simulink model "Dynamics_test"  (R2023b)
settings: Solver=FixedStepAuto  StartTime=0.0  StopTime=30  FixedStep=1e-4  RelTol=1e-3
values from neighbouring files (symbols this model uses):
  aircraft_b = 2    [initial.m]
  aircraft_c = 0.275    [initial.m]
  aircraft_mass = 6.031    [initial.m]
  c1 = ((Iyy - Izz)*Izz - Ixz*Ixz)/sigma    (= -0.404494382022)    [initial.m]
  c2 = ((Ixx - Iyy + Izz)*Ixz)/sigma    (= 0)    [initial.m]
  c3 = Izz/sigma    (= 3.74531835206)    [initial.m]
  c4 = Ixz/sigma    (= 0)    [initial.m]
  c5 = (Izz - Ixx)/Iyy    (= 0.404494382022)    [initial.m]
  c6 = Ixz/Iyy    (= 0)    [initial.m]
  c7 = 1/Iyy    (= 3.74531835206)    [initial.m]
  c8 = (Ixx*(Ixx - Iyy) + Ixz*Ixz)/sigma    (= 0)    [initial.m]
  c9 = Ixx/sigma    (= 2.66666666667)    [initial.m]
  CD_fuselage = 0.027    [initial.m]
  CdDa = 0.092132    [initial.m]
  CdDe = 0.016043    [initial.m]
  CdDr = 0.0097403    [initial.m]
  CDmin = 0.06047    [initial.m]
  CL0 = 0.81857    [initial.m]
  CL_CDmin = 0.4806    [initial.m]
  CLa = 4.09127    [initial.m]
  CLa_dot = 0    [initial.m]
  Clb = -0.00161    [initial.m]
  ClDa = 0.286593    [initial.m]
  CLDa = -0.85291    [initial.m]
  CLDe = 0.50787    [initial.m]
  ClDr = 0.013407    [initial.m]
  Clp = -0.47584    [initial.m]
  CLq = 7.31097    [initial.m]
  Clr = 0.27153    [initial.m]
  Cm0 = 0.00763    [initial.m]
  Cma = -1.76966    [initial.m]
  CmDe = -1.83747    [initial.m]
  Cmq = -19.22663    [initial.m]
  Cnb = 0.0918    [initial.m]
  CnDa = 0.0049274    [initial.m]
  CnDr = -0.067036    [initial.m]
  Cnp = -0.13267    [initial.m]
  Cnr = -0.08829    [initial.m]
  CYb = -0.00157    [initial.m]
  CYDr = 0.128915    [initial.m]
  CYp = -0.00157    [initial.m]
  CYr = 0.18368    [initial.m]
  F_T = C_T*rho*n_trim^2*PropDiameter^4    [initial.m]
  g = 9.8060    (= 9.806)    [initial.m]
  init_aileron = 0    [initial.m]
  init_alpha = alpha_trim    (= 0)    [initial.m]
  init_beta = atan(init_v/init_V)    [initial.m]
  init_elevator = elevator_trim    (= 0)    [initial.m]
  init_h = 10    [initial.m]
  init_p = 0    [initial.m]
  init_phi = 0    [initial.m]
  init_psi = 0    [initial.m]
  init_q = 0    [initial.m]
  init_r = 0    [initial.m]
  init_rudder = 0    [initial.m]
  init_theta = init_alpha    (= 0)    [initial.m]
  init_u = Vb(1)    [initial.m]
  init_v = Vb(2)    [initial.m]
  init_w = Vb(3)    [initial.m]
  init_x = 0    [initial.m]
  init_y = 0    [initial.m]
  K = 0.1328    [initial.m]
  Max_RPM = 10000    [initial.m]
  PropDiameter = 0.3052    [initial.m]
  rho = 1.2250    (= 1.225)    [initial.m]
  rotor1_direction = 1    [initial.m]
  rotor2_direction = -1    [initial.m]
  rotor3_direction = -1    [initial.m]
  rotor4_direction = 1    [initial.m]
  rotor_arm1 = [0.375,0.375,0]    [initial.m]
  rotor_arm2 = [0.375,-0.375,0]    [initial.m]
  rotor_arm3 = [-0.375,-0.375,0]    [initial.m]
  rotor_arm4 = [-0.375,0.375,0]    [initial.m]
  RPM_init = 0    [initial.m]
  tilt1_init = lambda    [initial.m]
  tilt2_init = lambda    [initial.m]
  tilt3_init = 0    [initial.m]
  tilt4_init = 0    [initial.m]
undefined symbols (not defined in the file or in its folder): linmodel, linmodel2
libraries: simulink_extras x14, aerolibasang x5, matrix_library x4
settings Model: Creator=admin  LastModifiedBy=admin

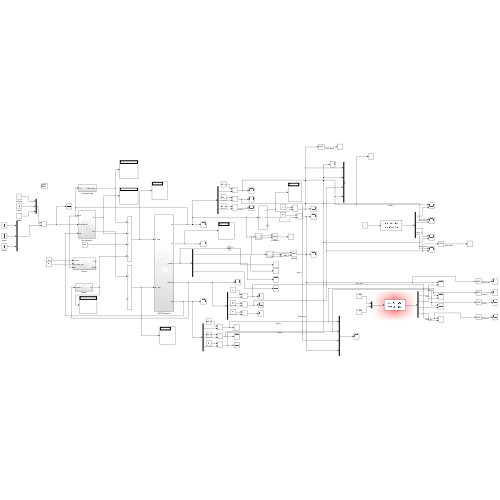
[thumbnail: Simulink's stored preview of the top-level diagram]
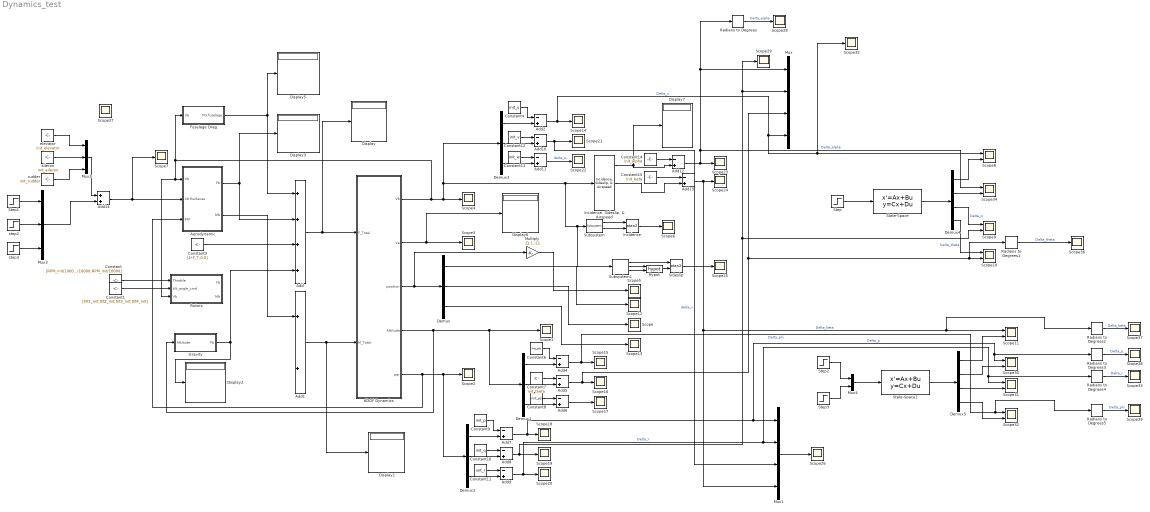
== system Dynamics_test ==
  6DOF Dynamics : Subsystem
  Add : Sum  Inputs=++++
  Add1 : Sum
  Add{2,4..13} (11 alike) : Sum  Inputs=-+
  Add14 : Sum
  Aerodynamic : Subsystem
  Constant : Constant  Value=[RPM_init/10000;RPM_init/10000;RPM_init/10000;RPM_init/10000]
  Constant1 : Constant  Value=[tilt1_init;tilt2_init;tilt3_init;tilt4_init]
  Constant10 : Constant  Value=init_q
  Constant11 : Constant  Value=init_r
  Constant12 : Constant  Value=init_v
  Constant13 : Constant  Value=init_w
  Constant14 : Constant  Value=init_alpha
  Constant15 : Constant  Value=init_beta
  Constant3 : Constant  Value=[4*F_T;0;0]
  Constant4 : Constant  Value=init_u
  Constant6 : Constant  Value=init_phi
  Constant7 : Constant  Value=init_theta
  Constant8 : Constant  Value=init_psi
  Constant9 : Constant  Value=init_p
  Demux{,1..3} (4 alike) : Demux  Outputs=3
  Demux4 : Demux
  Demux5 : Demux
  Display{,1..3,5..7} (7 alike) : Display
  Fuselage Drag : Subsystem
  Gravity : Subsystem
  Hypot : Math  Operator=hypot
  Incidence : Trigonometry  Operator=atan2
  "Incidence, Sideslip, & Airspeed" : aerolibasang/Incidence, Sideslip, & Airspeed
  Multiply : Gain  Gain=[1;1;-1]
  Mux : Mux
  Mux1 : Mux
  Mux2 : Mux  Inputs=3
  Mux3 : Mux  Inputs=3
  Mux4 : Mux  Inputs=2
  Radians to Degrees{,1..5} (6 alike) : simulink_extras/Transformations/Radians to Degrees
  Rotors : Subsystem
  Scope{,1..7,12..29,33,35..39} (32 alike) : Scope
  Scope{8..11,30..32,34} (8 alike) : Scope  NumInputPorts=2
  Sideslip : Trigonometry  Operator=atan2
  State-Space : StateSpace  A=linmodel.A  B=linmodel.B  C=linmodel.C  D=linmodel.D  InitialCondition=[0;0;0;0]
  State-Space1 : StateSpace  A=linmodel2.A  B=linmodel2.B  C=linmodel2.C  D=linmodel2.D  InitialCondition=[0;0;0;0]
  Step{,1..3} (4 alike) : Step  After=0  SampleTime=0
  Subsystem : aerolibasang/Incidence, Sideslip, & Airspeed/Subsystem  SystemSampleTime=-1  VariantActivationTime=update diagram  AllowFlexibleInterface=on  Latency=0  AutoFrameSizeCalculation=off
  Subsystem1 : aerolibasang/Incidence, Sideslip, & Airspeed/Subsystem1  SystemSampleTime=-1  VariantActivationTime=update diagram  AllowFlexibleInterface=on  Latency=0  AutoFrameSizeCalculation=off
  aileron : Constant  Value=init_aileron
  elevator : Constant  Value=init_elevator
  rudder : Constant  Value=init_rudder
  step2 : Step  After=0  SampleTime=0
  step3 : Step  After=deg2rad(1)  SampleTime=0
  wires:
  Add/1 -> 6DOF Dynamics/1(F_Total), Display/1
  Add1/1 -> 6DOF Dynamics/2(M_Total), Display1/1
  6DOF Dynamics/4(Attitude) -> Gravity/1(Attitude), Demux1/1, Scope1/1
  6DOF Dynamics/2(Ve) -> Display6/1, Scope3/1
  Demux/2 -> Scope/1
  Demux/1 -> Scope12/1
  Constant/1 -> Rotors/1(Throttle)
  Aerodynamic/2(Mb) -> Add1/1
  Constant1/1 -> Rotors/2(tilt_angle_cmd)
  Demux/3 -> Scope13/1
  Gravity/1(Fb) -> Add/4, Display2/1
  Aerodynamic/1(Fb) -> Display3/1, Add/2
  Fuselage Drag/1(FD,fuselage) -> Display5/1, Add/1
  6DOF Dynamics/3(position) -> Multiply/1, Demux/1
  Multiply/1 -> Scope5/1
  Constant3/1 -> Add/3
  Demux1/1 -> Add4/2
  Constant6/1 -> Add4/1
  Demux1/2 -> Add5/2
  Constant7/1 -> Add5/1
  Demux1/3 -> Add6/2
  Constant8/1 -> Add6/1
  Add4/1 -> Radians to Degrees5/1, Scope32/1, Scope15/1  "Delta_phi"
  Add5/1 -> Radians to Degrees1/1, Scope10/2, Mux/3, Scope16/1
  Add6/1 -> Scope17/1
  Add9/1 -> Radians to Degrees4/1, Scope31/1, Mux1/2, Scope20/1  "Delta_r"
  Constant11/1 -> Add9/1
  Constant9/1 -> Add7/1
  Add7/1 -> Radians to Degrees3/1, Scope30/1, Mux1/1, Scope18/1  "Delta_p"
  6DOF Dynamics/5(pqr) -> Aerodynamic/3(pqr), Demux2/1, Scope2/1
  Constant10/1 -> Add8/1
  Demux2/2 -> Add8/2
  Demux2/1 -> Add7/2
  Demux2/3 -> Add9/2
  Add11/1 -> Scope22/1  "delta_w"
  Constant13/1 -> Add11/1
  Constant4/1 -> Add2/1
  Add2/1 -> Scope35/1, Scope8/1, Mux/4, Scope14/1  "Delta_u"
  Constant12/1 -> Add10/1
  Demux3/2 -> Add10/2
  Demux3/1 -> Add2/2
  Demux3/3 -> Add11/2
  Constant14/1 -> Add12/1
  Add12/1 -> Scope34/1, Mux/1, Radians to Degrees/1, Scope23/1  "Delta_alpha"
  "Incidence, Sideslip, & Airspeed"/1 -> Display7/1, Add12/2
  Constant15/1 -> Add13/1
  "Incidence, Sideslip, & Airspeed"/2 -> Add13/2
  Add8/1 -> Scope9/2, Mux/2, Scope29/1, Scope19/1
  Add10/1 -> Mux1/3, Scope21/1  "delta_v"
  Add13/1 -> Radians to Degrees2/1, Scope11/1, Mux1/4, Scope24/1  "Delta_beta"
  Mux1/1 -> Scope26/1
  Add14/1 -> Scope7/1, Aerodynamic/2(CtrlSurfaces)
  Mux2/1 -> Add14/1
  rudder/1 -> Mux2/3
  aileron/1 -> Mux2/2
  elevator/1 -> Mux2/1
  Subsystem/2 -> Incidence/2
  Subsystem/1 -> Incidence/1
  Incidence/1 -> Scope6/1
  State-Space/1 -> Demux4/1
  Demux4/1 -> Scope8/2
  Step/1 -> State-Space/1
  step3/1 -> Mux3/3
  step2/1 -> Mux3/2
  Step1/1 -> Mux3/1
  Mux3/1 -> Add14/2
  Demux4/2 -> Scope34/2
  Demux4/3 -> Scope9/1  "Delta_q"
  Demux4/4 -> Scope10/1  "Delta_theta"
  Subsystem1/3 -> Hypot/2
  6DOF Dynamics/1(Vb) -> Fuselage Drag/1(Vb), Rotors/3(Vb), Aerodynamic/1(Vb), Demux3/1, Subsystem1/1, Subsystem/1, "Incidence, Sideslip, & Airspeed"/1, Scope4/1
  Hypot/1 -> Sideslip/2
  Subsystem1/2 -> Hypot/1
  Sideslip/1 -> Scope25/1
  Subsystem1/1 -> Sideslip/1
  State-Space1/1 -> Demux5/1
  Demux5/2 -> Scope30/2
  Demux5/3 -> Scope31/2
  Demux5/4 -> Scope32/2
  Step2/1 -> Mux4/1
  Step3/1 -> Mux4/2
  Mux4/1 -> State-Space1/1
  Demux5/1 -> Scope11/2
  Radians to Degrees/1 -> Scope28/1  "Delta_alpha"
  Radians to Degrees1/1 -> Scope36/1  "Delta_theta"
  Radians to Degrees2/1 -> Scope37/1  "Delta_beta"
  Radians to Degrees3/1 -> Scope38/1  "Delta_p"
  Radians to Degrees4/1 -> Scope33/1  "Delta_r"
  Radians to Degrees5/1 -> Scope39/1  "Delta_phi"

== system Dynamics_test/6DOF Dynamics ==
  F_Total : Inport
  M_Total : Inport  Port=2
  Attitude_Function : Subsystem
  Display : Display
  Force_Function : Subsystem
  Integrator : Integrator  InitialCondition=[init_u;init_v;init_w]
  Integrator1 : Integrator  InitialCondition=[init_phi;init_theta;init_psi]  WrapState=on
  Integrator2 : Integrator  InitialCondition=[init_x;init_y;-init_h]
  Integrator3 : Integrator  InitialCondition=[init_p;init_q;init_r]
  MatrixMultiply : Product  Multiplication=Matrix(*)
  Matrix_gb : Subsystem
  Moment_Function : Subsystem
  Transpose : Math  Operator=transpose
  Vb : Outport
  Ve : Outport  Port=2
  position : Outport  Port=3
  Attitude : Outport  Port=4
  pqr : Outport  Port=5
  wires:
  M_Total/1 -> Moment_Function/1(M_Total)
  Moment_Function/1(dot_pqr) -> Integrator3/1
  Integrator3/1 -> Force_Function/3(pqr), Attitude_Function/1(pqr), Moment_Function/2(pqr), pqr/1
  F_Total/1 -> Force_Function/2(F_Total)
  Force_Function/1(dot_Vb) -> Integrator/1
  Attitude_Function/1(dot_attitude) -> Integrator1/1
  Integrator1/1 -> Matrix_gb/1(Attitude), Attitude_Function/2(attitude), Attitude/1
  Matrix_gb/1(Mgb) -> Display/1, Transpose/1
  Integrator/1 -> Vb/1, MatrixMultiply/2, Force_Function/1(Vb)
  Transpose/1 -> MatrixMultiply/1
  MatrixMultiply/1 -> Ve/1, Integrator2/1
  Integrator2/1 -> position/1

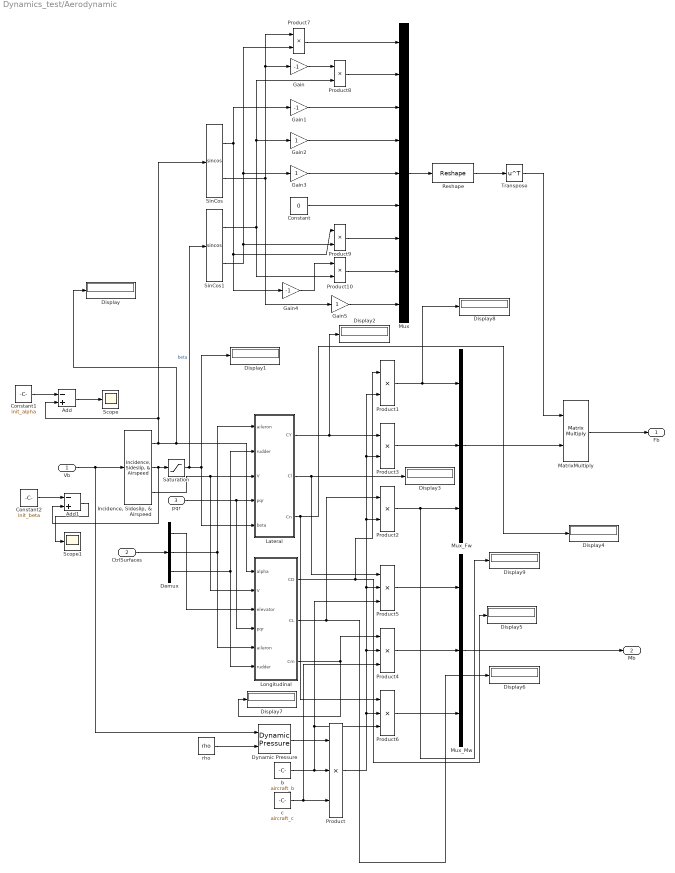
== system Dynamics_test/Aerodynamic ==
  Vb : Inport
  CtrlSurfaces : Inport  Port=2
  pqr : Inport  Port=3
  Add : Sum  Inputs=-+
  Add1 : Sum  Inputs=-+
  Constant : Constant  Value=0
  Constant1 : Constant  Value=init_alpha
  Constant2 : Constant  Value=init_beta
  Demux : Demux  Outputs=3
  Display{,1..9} (10 alike) : Display
  Dynamic Pressure : aerolibasang/Dynamic Pressure
  Gain : Gain  Gain=-1
  Gain1 : Gain  Gain=-1
  Gain2 : Gain
  Gain3 : Gain
  Gain4 : Gain  Gain=-1
  Gain5 : Gain
  "Incidence, Sideslip, & Airspeed" : aerolibasang/Incidence, Sideslip, & Airspeed
  Lateral : Subsystem
  Longitudinal : Subsystem
  MatrixMultiply : Product  Multiplication=Matrix(*)
  Mux : Mux  Inputs=9
  Mux_Fw : Mux  Inputs=3
  Mux_Mw : Mux  Inputs=3
  Product{,4..6} (4 alike) : Product  Inputs=3
  Product{1..3,7..10} (7 alike) : Product
  Reshape : Reshape  OutputDimensionality=Customize  OutputDimensions=[3,3]
  Saturation : Saturate  UpperLimit=14*pi/180  LowerLimit=-14*pi/180
  Scope : Scope
  Scope1 : Scope
  SinCos : Trigonometry  Operator=sincos
  SinCos1 : Trigonometry  Operator=sincos
  Transpose : Math  Operator=transpose
  b : Constant  Value=aircraft_b
  c : Constant  Value=aircraft_c
  rho : Constant  Value=rho
  Fb : Outport
  Mb : Outport  Port=2
  wires:
  Vb/1 -> "Incidence, Sideslip, & Airspeed"/1, Dynamic Pressure/1
  rho/1 -> Dynamic Pressure/2
  CtrlSurfaces/1 -> Demux/1
  Demux/2 -> Longitudinal/5(aileron), Lateral/1(aileron)
  Demux/3 -> Longitudinal/6(rudder), Lateral/2(rudder)
  "Incidence, Sideslip, & Airspeed"/3 -> Longitudinal/2(V), Lateral/3(V)
  pqr/1 -> Longitudinal/4(pqr), Lateral/4(pqr)
  "Incidence, Sideslip, & Airspeed"/2 -> Add1/2, Saturation/1
  "Incidence, Sideslip, & Airspeed"/1 -> Add/2, SinCos/1, Display/1, Longitudinal/1(alpha)
  Demux/1 -> Longitudinal/3(elevator)
  Dynamic Pressure/1 -> Product/1
  b/1 -> Product6/3, Product5/3, Product/2
  c/1 -> Product4/3, Product/3
  Longitudinal/1(CD) -> Display5/1, Product1/1
  Product/1 -> Product2/2, Product3/2, Product1/2, Product5/2, Product4/2, Product6/2
  Longitudinal/2(CL) -> Display6/1, Product2/1
  Lateral/1(CY) -> Display2/1, Product3/1
  Longitudinal/3(Cm) -> Product4/1, Display7/1
  Lateral/2(Cl) -> Product5/1, Display3/1
  Lateral/3(Cn) -> Product6/1, Display4/1
  Product3/1 -> Mux_Fw/2
  Product2/1 -> Display9/1, Mux_Fw/3
  Product1/1 -> Display8/1, Mux_Fw/1
  Mux_Fw/1 -> MatrixMultiply/2
  Product5/1 -> Mux_Mw/1
  Product4/1 -> Mux_Mw/2
  Product6/1 -> Mux_Mw/3
  SinCos/2 -> Gain5/1, Gain/1, Product7/1
  SinCos1/2 -> Product9/2, Gain3/1, Product7/2
  Gain/1 -> Product8/1
  SinCos1/1 -> Product10/2, Gain2/1, Product8/2
  SinCos/1 -> Gain1/1, Product9/1, Gain4/1
  Gain4/1 -> Product10/1
  Product7/1 -> Mux/1
  Product8/1 -> Mux/2
  Gain1/1 -> Mux/3
  Gain2/1 -> Mux/4
  Gain3/1 -> Mux/5
  Constant/1 -> Mux/6
  Product9/1 -> Mux/7
  Product10/1 -> Mux/8
  Gain5/1 -> Mux/9
  Mux/1 -> Reshape/1
  MatrixMultiply/1 -> Fb/1
  Reshape/1 -> Transpose/1
  Transpose/1 -> MatrixMultiply/1
  Mux_Mw/1 -> Mb/1
  Saturation/1 -> SinCos1/1, Display1/1, Lateral/5(beta)  "beta"
  Constant1/1 -> Add/1
  Add/1 -> Scope/1
  Constant2/1 -> Add1/1
  Add1/1 -> Scope1/1

== system Dynamics_test/Fuselage Drag ==
  Vb : Inport
  Add : Sum  Inputs=+++
  Constant : Constant  Value=CD_fuselage
  Demux : Demux  Outputs=3
  Gain : Gain  Gain=-1
  Product : Product
  Product1 : Product
  Sqrt : Sqrt
  Square : Math  Operator=square
  Square1 : Math  Operator=square
  Square2 : Math  Operator=square
  FD,fuselage : Outport
  wires:
  Vb/1 -> Product1/2, Demux/1
  Demux/1 -> Square/1
  Demux/2 -> Square1/1
  Demux/3 -> Square2/1
  Square/1 -> Add/1
  Square1/1 -> Add/2
  Square2/1 -> Add/3
  Add/1 -> Sqrt/1
  Sqrt/1 -> Product/2
  Constant/1 -> Product/1
  Product/1 -> Product1/1
  Product1/1 -> Gain/1
  Gain/1 -> FD,fuselage/1

== system Dynamics_test/Gravity ==
  Attitude : Inport
  Demux : Demux  Outputs=3
  Gain : Gain  Gain=-1
  Gain1 : Gain  Gain=aircraft_mass*g
  Mux : Mux  Inputs=3
  Product : Product
  Product1 : Product
  SinCos : Trigonometry  Operator=sincos
  SinCos1 : Trigonometry  Operator=sincos
  Fb : Outport
  wires:
  Attitude/1 -> Demux/1
  Demux/1 -> SinCos/1
  Demux/2 -> SinCos1/1
  SinCos1/2 -> Product/2, Product1/1
  SinCos/1 -> Product/1
  SinCos/2 -> Product1/2
  SinCos1/1 -> Gain/1
  Gain/1 -> Mux/1
  Product/1 -> Mux/2
  Product1/1 -> Mux/3
  Mux/1 -> Gain1/1
  Gain1/1 -> Fb/1

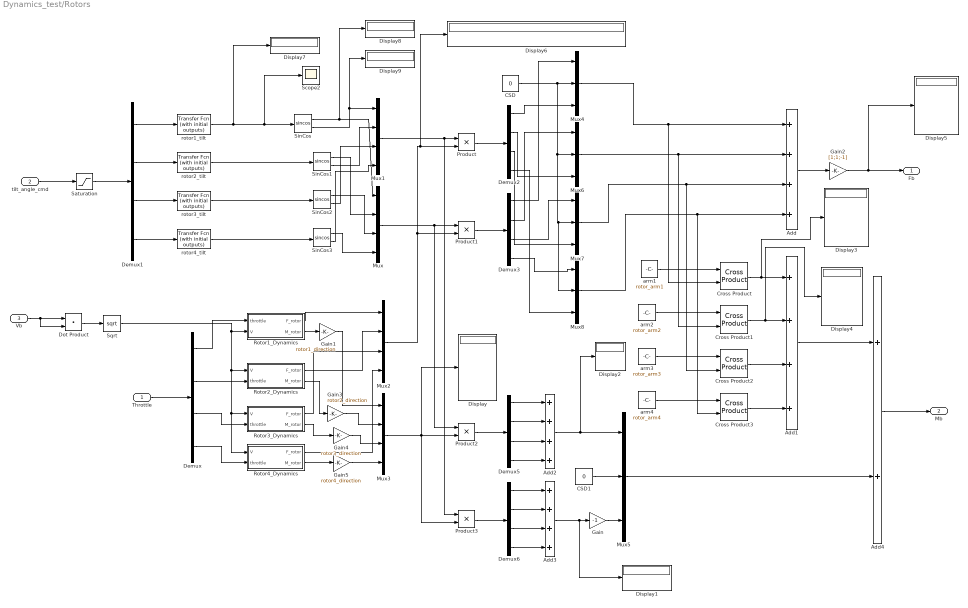
== system Dynamics_test/Rotors ==
  Throttle : Inport
  tilt_angle_cmd : Inport  Port=2
  Vb : Inport  Port=3
  Add{,1..3} (4 alike) : Sum  Inputs=++++
  Add4 : Sum
  CSD : Constant  Value=0
  CSD1 : Constant  Value=0
  Cross Product{,1..3} (4 alike) : matrix_library/Cross Product
  Demux{,1..3,5..6} (6 alike) : Demux
  Display{,1..9} (10 alike) : Display
  Dot Product : DotProduct  OutDataTypeStr=Inherit: Inherit via internal rule
  Gain : Gain  Gain=-1
  Gain1 : Gain  Gain=rotor1_direction
  Gain2 : Gain  Gain=[1;1;-1]
  Gain3 : Gain  Gain=rotor2_direction
  Gain4 : Gain  Gain=rotor3_direction
  Gain5 : Gain  Gain=rotor4_direction
  Mux{,1..3} (4 alike) : Mux
  Mux{4..8} (5 alike) : Mux  Inputs=3
  Product{,1..3} (4 alike) : Product
  Rotor1_Dynamics : Subsystem
  Rotor2_Dynamics : Subsystem
  Rotor3_Dynamics : Subsystem
  Rotor4_Dynamics : Subsystem
  Saturation : Saturate  UpperLimit=90*pi/180  LowerLimit=-90*pi/180
  Scope2 : Scope
  SinCos{,1..3} (4 alike) : Trigonometry  Operator=sincos
  Sqrt : Sqrt
  arm1 : Constant  Value=rotor_arm1
  arm2 : Constant  Value=rotor_arm2
  arm3 : Constant  Value=rotor_arm3
  arm4 : Constant  Value=rotor_arm4
  rotor1_tilt : simulink_extras/Additional Linear/Transfer Fcn (with initial outputs)  N=[1]  D="[0.1  1]"  Y0=tilt1_init  U0=tilt1_init
  rotor2_tilt : simulink_extras/Additional Linear/Transfer Fcn (with initial outputs)  N=[1]  D="[0.1  1]"  Y0=tilt2_init  U0=tilt2_init
  rotor3_tilt : simulink_extras/Additional Linear/Transfer Fcn (with initial outputs)  N=[1]  D="[0.1  1]"  Y0=tilt3_init  U0=tilt3_init
  rotor4_tilt : simulink_extras/Additional Linear/Transfer Fcn (with initial outputs)  N=[1]  D="[0.1  1]"  Y0=tilt4_init  U0=tilt4_init
  Fb : Outport
  Mb : Outport  Port=2
  wires:
  Throttle/1 -> Demux/1
  Demux/1 -> Rotor1_Dynamics/1(throttle)
  Demux1/1 -> rotor1_tilt/1
  Demux1/2 -> rotor2_tilt/1
  Demux1/3 -> rotor3_tilt/1
  Demux1/4 -> rotor4_tilt/1
  tilt_angle_cmd/1 -> Saturation/1
  Saturation/1 -> Demux1/1
  rotor1_tilt/1 -> Display7/1, SinCos/1, Scope2/1
  rotor2_tilt/1 -> SinCos1/1
  rotor3_tilt/1 -> SinCos2/1
  rotor4_tilt/1 -> SinCos3/1
  SinCos/1 -> Display8/1, Mux/1
  SinCos1/1 -> Mux/2
  SinCos2/1 -> Mux/3
  SinCos3/1 -> Mux/4
  SinCos/2 -> Display9/1, Mux1/1
  SinCos1/2 -> Mux1/2
  SinCos2/2 -> Mux1/3
  SinCos3/2 -> Mux1/4
  Rotor1_Dynamics/1(F_rotor) -> Mux2/1
  Mux2/1 -> Product1/2, Display6/1, Product/2
  Product/1 -> Demux2/1
  Product1/1 -> Demux3/1
  Add/1 -> Gain2/1
  Mux3/1 -> Product3/2, Display/1, Product2/2
  Mux/1 -> Product2/1, Product1/1
  Product2/1 -> Demux5/1
  Product3/1 -> Demux6/1
  Demux5/1 -> Add2/1
  Demux5/2 -> Add2/2
  Demux5/3 -> Add2/3
  Demux5/4 -> Add2/4
  Demux6/1 -> Add3/1
  Demux6/2 -> Add3/2
  Demux6/3 -> Add3/3
  Demux6/4 -> Add3/4
  Add3/1 -> Display1/1, Gain/1
  Add2/1 -> Display2/1, Mux5/1
  CSD1/1 -> Mux5/2
  CSD/1 -> Mux8/2, Mux7/2, Mux6/2, Mux4/2
  Mux4/1 -> Cross Product/2, Add/1
  Mux7/1 -> Add/3, Cross Product2/2
  Mux8/1 -> Cross Product3/2, Add/4
  arm1/1 -> Cross Product/1
  arm2/1 -> Cross Product1/1
  Mux6/1 -> Add/2, Cross Product1/2
  arm3/1 -> Cross Product2/1
  arm4/1 -> Cross Product3/1
  Cross Product/1 -> Display3/1, Add1/1
  Cross Product1/1 -> Display4/1, Add1/2
  Cross Product2/1 -> Add1/3
  Cross Product3/1 -> Add1/4
  Add1/1 -> Add4/1
  Mux5/1 -> Add4/2
  Add4/1 -> Mb/1
  Gain2/1 -> Display5/1, Fb/1
  Vb/1 -> Dot Product/2, Dot Product/1
  Dot Product/1 -> Sqrt/1
  Sqrt/1 -> Rotor4_Dynamics/1(V), Rotor3_Dynamics/1(V), Rotor2_Dynamics/1(V), Rotor1_Dynamics/2(V)
  Rotor1_Dynamics/2(M_rotor) -> Gain1/1
  Demux/2 -> Rotor2_Dynamics/2(throttle)
  Rotor2_Dynamics/1(F_rotor) -> Mux2/2
  Rotor2_Dynamics/2(M_rotor) -> Gain3/1
  Demux/3 -> Rotor3_Dynamics/2(throttle)
  Rotor3_Dynamics/1(F_rotor) -> Mux2/3
  Rotor3_Dynamics/2(M_rotor) -> Gain4/1
  Demux/4 -> Rotor4_Dynamics/2(throttle)
  Rotor4_Dynamics/1(F_rotor) -> Mux2/4
  Rotor4_Dynamics/2(M_rotor) -> Gain5/1
  Demux3/1 -> Mux4/1
  Demux3/2 -> Mux6/1
  Demux3/3 -> Mux7/1
  Demux3/4 -> Mux8/1
  Demux2/1 -> Mux4/3
  Demux2/2 -> Mux6/3
  Demux2/3 -> Mux7/3
  Demux2/4 -> Mux8/3
  Gain/1 -> Mux5/3
  Gain1/1 -> Mux3/1
  Gain3/1 -> Mux3/2
  Gain4/1 -> Mux3/3
  Gain5/1 -> Mux3/4
  Mux1/1 -> Product3/1, Product/1

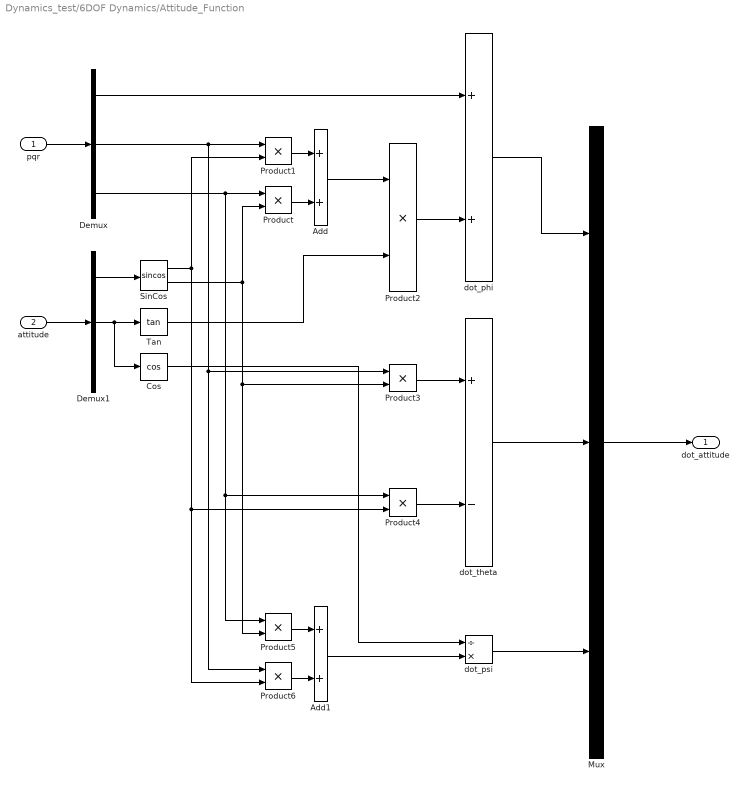
== system Dynamics_test/6DOF Dynamics/Attitude_Function ==
  pqr : Inport
  attitude : Inport  Port=2
  Add : Sum
  Add1 : Sum
  Cos : Trigonometry  Operator=cos
  Demux : Demux  Outputs=3
  Demux1 : Demux  Outputs=3
  Mux : Mux  Inputs=3
  Product{,1..6} (7 alike) : Product
  SinCos : Trigonometry  Operator=sincos
  Tan : Trigonometry  Operator=tan
  dot_phi : Sum
  dot_psi : Product  Inputs=/*
  dot_theta : Sum  Inputs=+-
  dot_attitude : Outport
  wires:
  pqr/1 -> Demux/1
  attitude/1 -> Demux1/1
  Demux1/2 -> Cos/1, Tan/1
  Demux1/1 -> SinCos/1
  Demux/3 -> Product5/1, Product4/1, Product/1
  SinCos/2 -> Product5/2, Product3/2, Product/2
  SinCos/1 -> Product4/2, Product6/2, Product1/2
  Demux/2 -> Product6/1, Product3/1, Product1/1
  Product/1 -> Add/2
  Product1/1 -> Add/1
  Tan/1 -> Product2/2
  Add/1 -> Product2/1
  Demux/1 -> dot_phi/1
  Product2/1 -> dot_phi/2
  Product3/1 -> dot_theta/1
  Product4/1 -> dot_theta/2
  Product5/1 -> Add1/1
  Product6/1 -> Add1/2
  Cos/1 -> dot_psi/1
  Add1/1 -> dot_psi/2
  dot_psi/1 -> Mux/3
  dot_theta/1 -> Mux/2
  dot_phi/1 -> Mux/1
  Mux/1 -> dot_attitude/1

== system Dynamics_test/6DOF Dynamics/Force_Function ==
  Vb : Inport
  F_Total : Inport  Port=2
  pqr : Inport  Port=3
  Demux : Demux  Outputs=3
  Demux1 : Demux  Outputs=3
  Demux2 : Demux  Outputs=3
  Gain : Gain  Gain=1/aircraft_mass
  Mux : Mux  Inputs=3
  Product{,1..5} (6 alike) : Product
  dot_u : Sum  Inputs=++-
  dot_v : Sum  Inputs=++-
  dot_w : Sum  Inputs=++-
  dot_Vb : Outport
  wires:
  Vb/1 -> Demux/1
  pqr/1 -> Demux1/1
  F_Total/1 -> Gain/1
  Demux/2 -> Product5/1, Product/1
  Demux1/3 -> Product2/2, Product/2
  Demux/3 -> Product3/1, Product1/1
  Demux1/2 -> Product4/2, Product1/2
  Gain/1 -> Demux2/1
  Product1/1 -> dot_u/3
  Product/1 -> dot_u/2
  Demux2/1 -> dot_u/1
  Demux/1 -> Product4/1, Product2/1
  Demux1/1 -> Product5/2, Product3/2
  Product3/1 -> dot_v/2
  Demux2/2 -> dot_v/1
  Product2/1 -> dot_v/3
  Product4/1 -> dot_w/2
  Product5/1 -> dot_w/3
  Demux2/3 -> dot_w/1
  dot_u/1 -> Mux/1
  dot_v/1 -> Mux/2
  dot_w/1 -> Mux/3
  Mux/1 -> dot_Vb/1

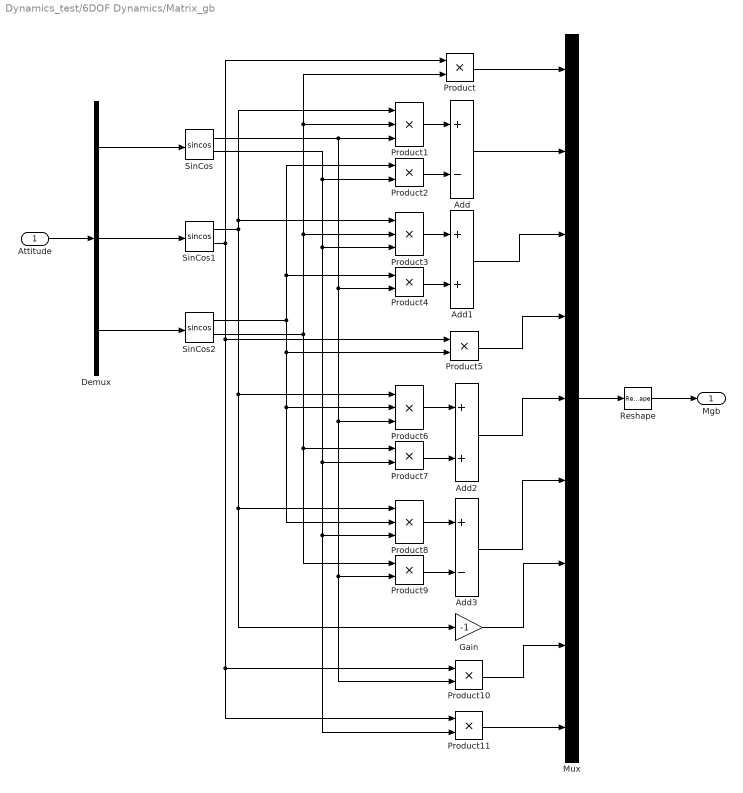
== system Dynamics_test/6DOF Dynamics/Matrix_gb ==
  Attitude : Inport
  Add : Sum  Inputs=+-
  Add1 : Sum
  Add2 : Sum
  Add3 : Sum  Inputs=+-
  Demux : Demux  Outputs=3
  Gain : Gain  Gain=-1
  Mux : Mux  Inputs=9
  Product{,2,4..5,7,9..11} (8 alike) : Product
  Product{1,3,6,8} (4 alike) : Product  Inputs=3
  Reshape : Reshape  OutputDimensionality=Customize  OutputDimensions=[3,3]
  SinCos : Trigonometry  Operator=sincos
  SinCos1 : Trigonometry  Operator=sincos
  SinCos2 : Trigonometry  Operator=sincos
  Mgb : Outport
  wires:
  Attitude/1 -> Demux/1
  Demux/1 -> SinCos/1
  Demux/2 -> SinCos1/1
  Demux/3 -> SinCos2/1
  SinCos1/2 -> Product/1, Product11/1, Product10/1, Product5/1
  SinCos2/2 -> Product3/2, Product/2, Product1/2, Product9/1, Product7/1
  SinCos1/1 -> Product3/1, Product1/1, Product6/1, Gain/1, Product8/1
  SinCos/1 -> Product10/2, Product9/2, Product6/3, Product4/2, Product1/3
  Product1/1 -> Add/1
  Product2/1 -> Add/2
  SinCos2/1 -> Product4/1, Product2/1, Product8/2, Product6/2, Product5/2
  SinCos/2 -> Product7/2, Product11/2, Product8/3, Product3/3, Product2/2
  Product3/1 -> Add1/1
  Product4/1 -> Add1/2
  Product6/1 -> Add2/1
  Product7/1 -> Add2/2
  Product8/1 -> Add3/1
  Product9/1 -> Add3/2
  Product/1 -> Mux/1
  Add/1 -> Mux/2
  Add1/1 -> Mux/3
  Product5/1 -> Mux/4
  Add2/1 -> Mux/5
  Add3/1 -> Mux/6
  Gain/1 -> Mux/7
  Product10/1 -> Mux/8
  Product11/1 -> Mux/9
  Mux/1 -> Reshape/1
  Reshape/1 -> Mgb/1

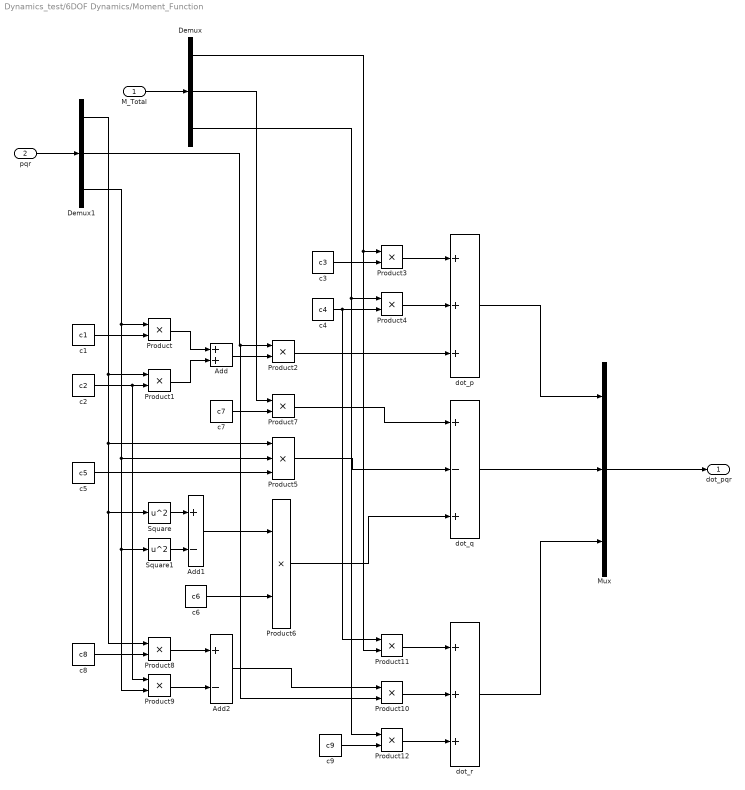
== system Dynamics_test/6DOF Dynamics/Moment_Function ==
  M_Total : Inport
  pqr : Inport  Port=2
  Add : Sum
  Add1 : Sum  Inputs=+-
  Add2 : Sum  Inputs=+-
  Demux : Demux  Outputs=3
  Demux1 : Demux  Outputs=3
  Mux : Mux  Inputs=3
  Product{,1..4,6..12} (12 alike) : Product
  Product5 : Product  Inputs=3
  Square : Math  Operator=square
  Square1 : Math  Operator=square
  c1 : Constant  Value=c1
  c2 : Constant  Value=c2
  c3 : Constant  Value=c3
  c4 : Constant  Value=c4
  c5 : Constant  Value=c5
  c6 : Constant  Value=c6
  c7 : Constant  Value=c7
  c8 : Constant  Value=c8
  c9 : Constant  Value=c9
  dot_p : Sum  Inputs=+++
  dot_q : Sum  Inputs=+-+
  dot_r : Sum  Inputs=+++
  dot_pqr : Outport
  wires:
  M_Total/1 -> Demux/1
  pqr/1 -> Demux1/1
  c1/1 -> Product/2
  Demux1/3 -> Product9/2, Square1/1, Product5/2, Product/1
  c2/1 -> Product9/1, Product1/2
  Demux1/1 -> Square/1, Product8/1, Product5/1, Product1/1
  Product1/1 -> Add/2
  Product/1 -> Add/1
  Add/1 -> Product2/2
  Demux1/2 -> Product10/2, Product2/1
  c3/1 -> Product3/2
  Demux/1 -> Product3/1, Product11/2
  Demux/3 -> Product4/1, Product12/1
  c4/1 -> Product11/1, Product4/2
  Product2/1 -> dot_p/3
  Product4/1 -> dot_p/2
  Product3/1 -> dot_p/1
  c5/1 -> Product5/3
  Square/1 -> Add1/1
  Square1/1 -> Add1/2
  Add1/1 -> Product6/1
  c6/1 -> Product6/2
  c7/1 -> Product7/2
  Demux/2 -> Product7/1
  Product7/1 -> dot_q/1
  Product5/1 -> dot_q/2
  Product6/1 -> dot_q/3
  c8/1 -> Product8/2
  Product8/1 -> Add2/1
  Product9/1 -> Add2/2
  Add2/1 -> Product10/1
  c9/1 -> Product12/2
  Product11/1 -> dot_r/1
  Product10/1 -> dot_r/2
  Product12/1 -> dot_r/3
  dot_q/1 -> Mux/2
  dot_r/1 -> Mux/3
  dot_p/1 -> Mux/1
  Mux/1 -> dot_pqr/1

== system Dynamics_test/Aerodynamic/Lateral ==
  aileron : Inport
  rudder : Inport  Port=2
  V : Inport  Port=3
  pqr : Inport  Port=4
  beta : Inport  Port=5
  Coff_CY : Subsystem
  Coff_Cl : Subsystem
  Subsystem : Subsystem
  CY : Outport
  Cl : Outport  Port=2
  Cn : Outport  Port=3
  wires:
  beta/1 -> Subsystem/1(beta), Coff_Cl/1(beta), Coff_CY/1(beta)
  rudder/1 -> Coff_Cl/3(rudder), Subsystem/3(rudder), Coff_CY/2(Rudder)
  pqr/1 -> Subsystem/4(pqr), Coff_Cl/5(pqr), Coff_CY/3(pqr)
  V/1 -> Subsystem/5(V), Coff_Cl/4(V), Coff_CY/4(V)
  Coff_CY/1(CY) -> CY/1
  aileron/1 -> Subsystem/2(aileron), Coff_Cl/2(aileron)
  Coff_Cl/1(Cl) -> Cl/1
  Subsystem/1(Cn) -> Cn/1

== system Dynamics_test/Aerodynamic/Longitudinal ==
  alpha : Inport
  V : Inport  Port=2
  elevator : Inport  Port=3
  pqr : Inport  Port=4
  aileron : Inport  Port=5
  rudder : Inport  Port=6
  Coff_D : Subsystem
  Coff_L : Subsystem
  Gain : Gain  Gain=-1
  Saturation : Saturate  UpperLimit=14*pi/180  LowerLimit=-14*pi/180
  Subsystem : Subsystem
  Transfer Fcn : TransferFcn  Numerator=[1 0]  Denominator=[0.1 1]
  CD : Outport
  CL : Outport  Port=2
  Cm : Outport  Port=3
  wires:
  aileron/1 -> Coff_L/6(aileron), Coff_D/2(aileron)
  rudder/1 -> Coff_D/3(rudder)
  elevator/1 -> Subsystem/2(elevator), Coff_L/3(elevator), Coff_D/4(elevator)
  Coff_D/1(CD) -> CD/1
  alpha/1 -> Saturation/1
  Saturation/1 -> Transfer Fcn/1, Subsystem/1(alpha), Coff_L/1(alpha)
  Transfer Fcn/1 -> Coff_L/2(alpha_dot)
  pqr/1 -> Subsystem/3(pqr), Coff_L/4(pqr)
  V/1 -> Subsystem/4(V), Coff_L/5(V)
  Coff_L/1(CL) -> Coff_D/1(CL), Gain/1
  Subsystem/1(Cm) -> Cm/1
  Gain/1 -> CL/1

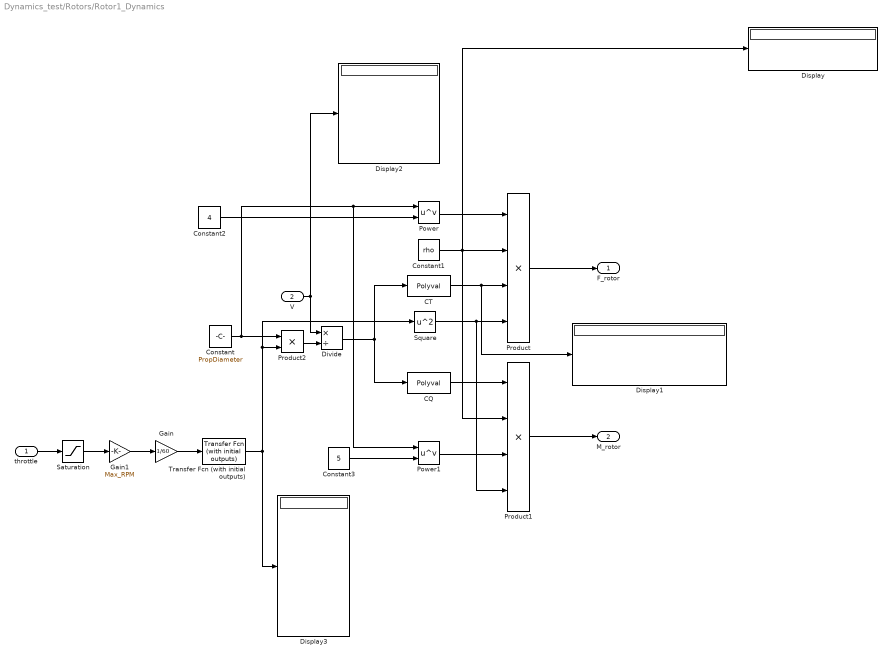
== system Dynamics_test/Rotors/Rotor1_Dynamics ==
  throttle : Inport
  V : Inport  Port=2
  CQ : Polyval  Coefs=[0.04280,-0.05046,0.005711,-0.003293, 0.007048]
  CT : Polyval  Coefs=[0.03338, -0.1265,-0.1210,0.1142]
  Constant : Constant  Value=PropDiameter
  Constant1 : Constant  Value=rho
  Constant2 : Constant  Value=4
  Constant3 : Constant  Value=5
  Display{,1..3} (4 alike) : Display
  Divide : Product  Inputs=*/
  Gain : Gain  Gain=1/60
  Gain1 : Gain  Gain=Max_RPM
  Power : Math  Operator=pow
  Power1 : Math  Operator=pow
  Product : Product  Inputs=4
  Product1 : Product  Inputs=4
  Product2 : Product
  Saturation : Saturate  UpperLimit=1  LowerLimit=0.01
  Square : Math  Operator=square
  Transfer Fcn (with initial outputs) : simulink_extras/Additional Linear/Transfer Fcn (with initial outputs)  N=[1]  D="[0.02  1]"  Y0=rotor_n  U0=rotor_n
  F_rotor : Outport
  M_rotor : Outport  Port=2
  wires:
  Gain/1 -> Transfer Fcn (with initial outputs)/1
  Saturation/1 -> Gain1/1
  throttle/1 -> Saturation/1
  Gain1/1 -> Gain/1
  Constant/1 -> Power1/1, Power/1, Product2/1
  Transfer Fcn (with initial outputs)/1 -> Display3/1, Square/1, Product2/2
  Product2/1 -> Divide/2
  V/1 -> Display2/1, Divide/1
  Divide/1 -> CQ/1, CT/1
  Constant2/1 -> Power/2
  Power/1 -> Product/1
  Constant1/1 -> Product1/2, Display/1, Product/2
  CT/1 -> Display1/1, Product/3
  Square/1 -> Product1/4, Product/4
  Product/1 -> F_rotor/1
  CQ/1 -> Product1/1
  Power1/1 -> Product1/3
  Constant3/1 -> Power1/2
  Product1/1 -> M_rotor/1

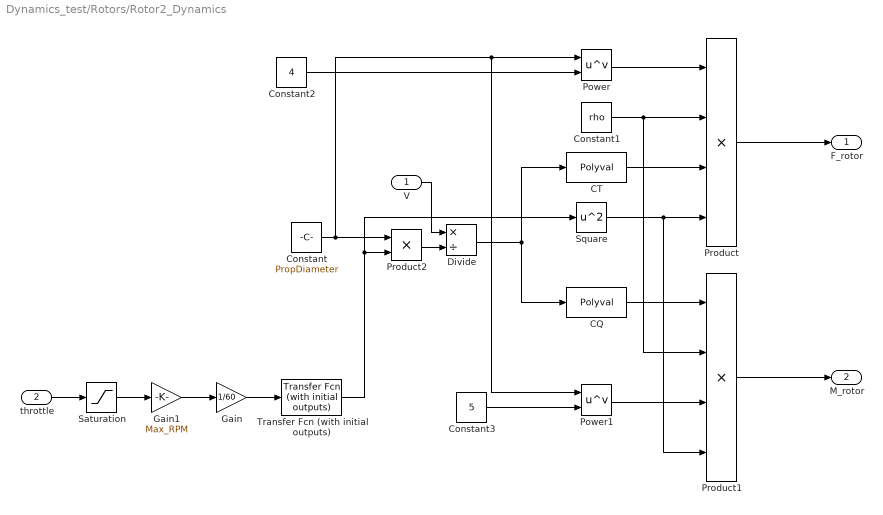
== system Dynamics_test/Rotors/Rotor2_Dynamics ==
  V : Inport
  throttle : Inport  Port=2
  CQ : Polyval  Coefs=[0.04280,-0.05046,0.005711,-0.003293, 0.007048]
  CT : Polyval  Coefs=[0.03338, -0.1265,-0.1210,0.1142]
  Constant : Constant  Value=PropDiameter
  Constant1 : Constant  Value=rho
  Constant2 : Constant  Value=4
  Constant3 : Constant  Value=5
  Divide : Product  Inputs=*/
  Gain : Gain  Gain=1/60
  Gain1 : Gain  Gain=Max_RPM
  Power : Math  Operator=pow
  Power1 : Math  Operator=pow
  Product : Product  Inputs=4
  Product1 : Product  Inputs=4
  Product2 : Product
  Saturation : Saturate  UpperLimit=1  LowerLimit=0.01
  Square : Math  Operator=square
  Transfer Fcn (with initial outputs) : simulink_extras/Additional Linear/Transfer Fcn (with initial outputs)  N=[1]  D="[0.02  1]"  Y0=rotor_n  U0=rotor_n
  F_rotor : Outport
  M_rotor : Outport  Port=2
  wires:
  Gain/1 -> Transfer Fcn (with initial outputs)/1
  Saturation/1 -> Gain1/1
  throttle/1 -> Saturation/1
  Gain1/1 -> Gain/1
  Constant/1 -> Power1/1, Power/1, Product2/1
  Transfer Fcn (with initial outputs)/1 -> Square/1, Product2/2
  Product2/1 -> Divide/2
  V/1 -> Divide/1
  Divide/1 -> CQ/1, CT/1
  Constant2/1 -> Power/2
  Power/1 -> Product/1
  Constant1/1 -> Product1/2, Product/2
  CT/1 -> Product/3
  Square/1 -> Product1/4, Product/4
  Product/1 -> F_rotor/1
  CQ/1 -> Product1/1
  Power1/1 -> Product1/3
  Constant3/1 -> Power1/2
  Product1/1 -> M_rotor/1

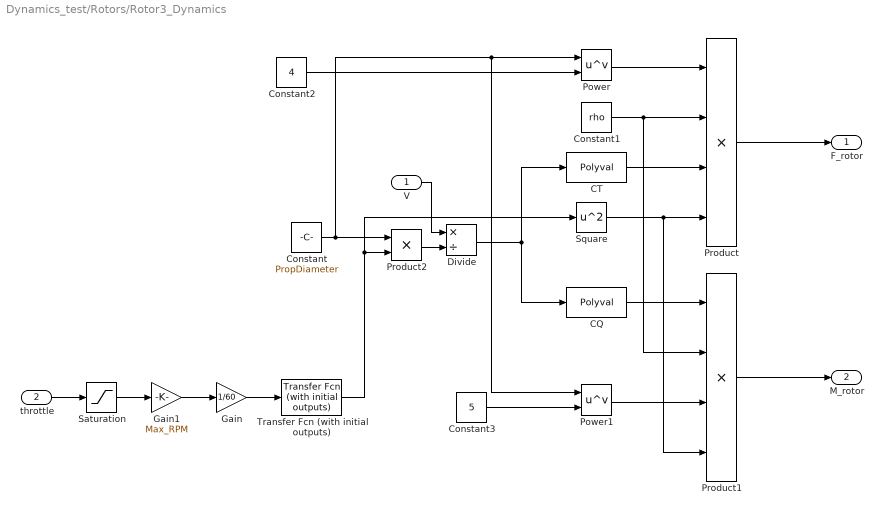
== system Dynamics_test/Rotors/Rotor3_Dynamics ==
  V : Inport
  throttle : Inport  Port=2
  CQ : Polyval  Coefs=[0.04280,-0.05046,0.005711,-0.003293, 0.007048]
  CT : Polyval  Coefs=[0.03338, -0.1265,-0.1210,0.1142]
  Constant : Constant  Value=PropDiameter
  Constant1 : Constant  Value=rho
  Constant2 : Constant  Value=4
  Constant3 : Constant  Value=5
  Divide : Product  Inputs=*/
  Gain : Gain  Gain=1/60
  Gain1 : Gain  Gain=Max_RPM
  Power : Math  Operator=pow
  Power1 : Math  Operator=pow
  Product : Product  Inputs=4
  Product1 : Product  Inputs=4
  Product2 : Product
  Saturation : Saturate  UpperLimit=1  LowerLimit=0.01
  Square : Math  Operator=square
  Transfer Fcn (with initial outputs) : simulink_extras/Additional Linear/Transfer Fcn (with initial outputs)  N=[1]  D="[0.02  1]"  Y0=rotor_n  U0=rotor_n
  F_rotor : Outport
  M_rotor : Outport  Port=2
  wires:
  Gain/1 -> Transfer Fcn (with initial outputs)/1
  Saturation/1 -> Gain1/1
  throttle/1 -> Saturation/1
  Gain1/1 -> Gain/1
  Constant/1 -> Power1/1, Power/1, Product2/1
  Transfer Fcn (with initial outputs)/1 -> Square/1, Product2/2
  Product2/1 -> Divide/2
  V/1 -> Divide/1
  Divide/1 -> CQ/1, CT/1
  Constant2/1 -> Power/2
  Power/1 -> Product/1
  Constant1/1 -> Product1/2, Product/2
  CT/1 -> Product/3
  Square/1 -> Product1/4, Product/4
  Product/1 -> F_rotor/1
  CQ/1 -> Product1/1
  Power1/1 -> Product1/3
  Constant3/1 -> Power1/2
  Product1/1 -> M_rotor/1

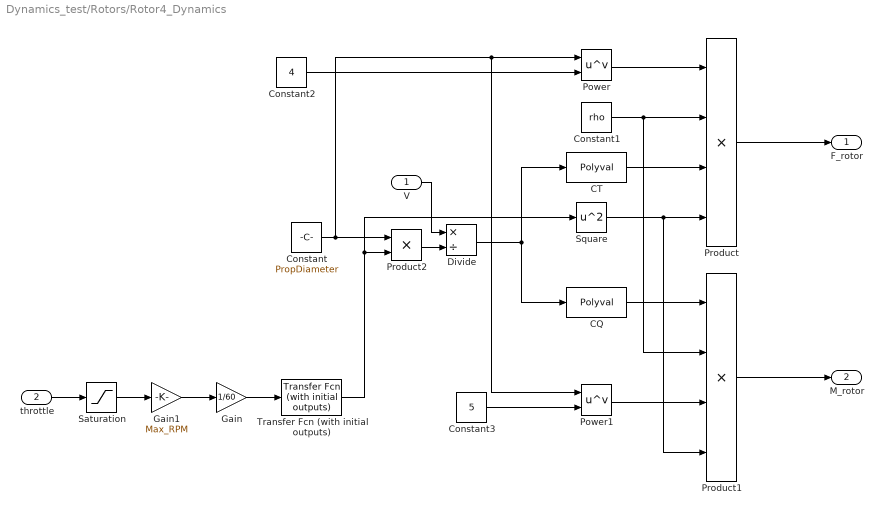
== system Dynamics_test/Rotors/Rotor4_Dynamics ==
  V : Inport
  throttle : Inport  Port=2
  CQ : Polyval  Coefs=[0.04280,-0.05046,0.005711,-0.003293, 0.007048]
  CT : Polyval  Coefs=[0.03338, -0.1265,-0.1210,0.1142]
  Constant : Constant  Value=PropDiameter
  Constant1 : Constant  Value=rho
  Constant2 : Constant  Value=4
  Constant3 : Constant  Value=5
  Divide : Product  Inputs=*/
  Gain : Gain  Gain=1/60
  Gain1 : Gain  Gain=Max_RPM
  Power : Math  Operator=pow
  Power1 : Math  Operator=pow
  Product : Product  Inputs=4
  Product1 : Product  Inputs=4
  Product2 : Product
  Saturation : Saturate  UpperLimit=1  LowerLimit=0.01
  Square : Math  Operator=square
  Transfer Fcn (with initial outputs) : simulink_extras/Additional Linear/Transfer Fcn (with initial outputs)  N=[1]  D="[0.02  1]"  Y0=rotor_n  U0=rotor_n
  F_rotor : Outport
  M_rotor : Outport  Port=2
  wires:
  Gain/1 -> Transfer Fcn (with initial outputs)/1
  Saturation/1 -> Gain1/1
  throttle/1 -> Saturation/1
  Gain1/1 -> Gain/1
  Constant/1 -> Power1/1, Power/1, Product2/1
  Transfer Fcn (with initial outputs)/1 -> Square/1, Product2/2
  Product2/1 -> Divide/2
  V/1 -> Divide/1
  Divide/1 -> CQ/1, CT/1
  Constant2/1 -> Power/2
  Power/1 -> Product/1
  Constant1/1 -> Product1/2, Product/2
  CT/1 -> Product/3
  Square/1 -> Product1/4, Product/4
  Product/1 -> F_rotor/1
  CQ/1 -> Product1/1
  Power1/1 -> Product1/3
  Constant3/1 -> Power1/2
  Product1/1 -> M_rotor/1

== system Dynamics_test/Aerodynamic/Lateral/Coff_CY ==
  beta : Inport
  Rudder : Inport  Port=2
  pqr : Inport  Port=3
  V : Inport  Port=4
  Add : Sum  Inputs=++++
  CYDr : Constant  Value=CYDr
  CYb : Constant  Value=CYb
  Product : Product
  Product1 : Product
  roll/yaw factors : Subsystem
  CY : Outport
  wires:
  CYb/1 -> Product/1
  beta/1 -> Product/2
  Add/1 -> CY/1
  Product/1 -> Add/1
  Rudder/1 -> Product1/1
  CYDr/1 -> Product1/2
  Product1/1 -> Add/2
  pqr/1 -> roll/yaw factors/1(pqr)
  V/1 -> roll/yaw factors/2(V)
  roll/yaw factors/1(CYp) -> Add/3
  roll/yaw factors/2(CYr) -> Add/4

== system Dynamics_test/Aerodynamic/Lateral/Coff_Cl ==
  beta : Inport
  aileron : Inport  Port=2
  rudder : Inport  Port=3
  V : Inport  Port=4
  pqr : Inport  Port=5
  Add : Sum  Inputs=+++++
  ClDa : Constant  Value=ClDa
  ClDr : Constant  Value=ClDr
  Clb : Constant  Value=Clb
  Product : Product
  Product1 : Product
  Product2 : Product
  roll/yaw factors : Subsystem
  Cl : Outport
  wires:
  beta/1 -> Product/2
  Clb/1 -> Product/1
  Product/1 -> Add/1
  ClDa/1 -> Product1/1
  aileron/1 -> Product1/2
  ClDr/1 -> Product2/1
  rudder/1 -> Product2/2
  Product1/1 -> Add/2
  Product2/1 -> Add/3
  pqr/1 -> roll/yaw factors/1(pqr)
  V/1 -> roll/yaw factors/2(V)
  roll/yaw factors/1(Clp) -> Add/4
  roll/yaw factors/2(Clr) -> Add/5
  Add/1 -> Cl/1

== system Dynamics_test/Aerodynamic/Lateral/Subsystem ==
  beta : Inport
  aileron : Inport  Port=2
  rudder : Inport  Port=3
  pqr : Inport  Port=4
  V : Inport  Port=5
  Add : Sum  Inputs=+++++
  CnDa : Constant  Value=CnDa
  CnDr : Constant  Value=CnDr
  Cnb : Constant  Value=Cnb
  Product : Product
  Product1 : Product
  Product2 : Product
  roll/yaw factors : Subsystem
  Cn : Outport
  wires:
  beta/1 -> Product/2
  Cnb/1 -> Product/1
  aileron/1 -> Product1/2
  CnDa/1 -> Product1/1
  rudder/1 -> Product2/2
  CnDr/1 -> Product2/1
  Product/1 -> Add/1
  Product1/1 -> Add/2
  Product2/1 -> Add/3
  Add/1 -> Cn/1
  pqr/1 -> roll/yaw factors/1(pqr)
  V/1 -> roll/yaw factors/2(V)
  roll/yaw factors/1(Cnp) -> Add/4
  roll/yaw factors/2(Cnr) -> Add/5

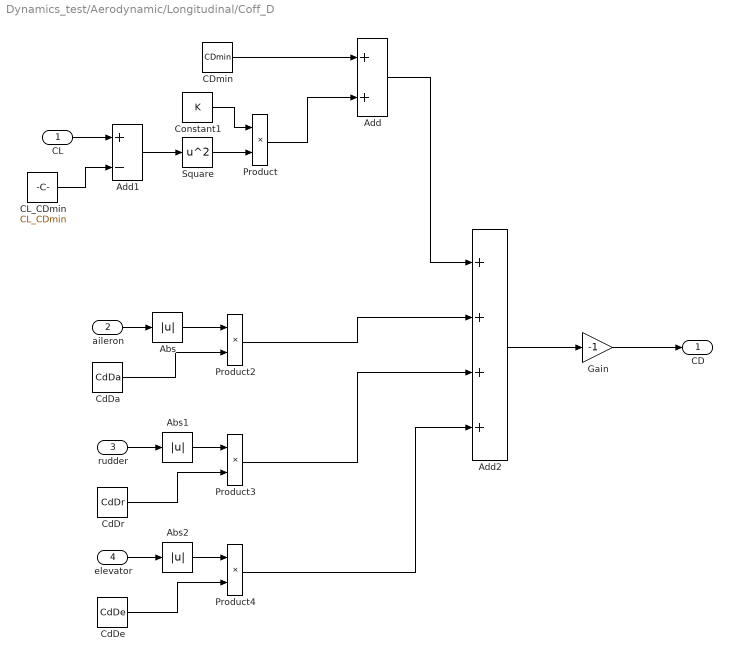
== system Dynamics_test/Aerodynamic/Longitudinal/Coff_D ==
  CL : Inport
  aileron : Inport  Port=2
  rudder : Inport  Port=3
  elevator : Inport  Port=4
  Abs : Abs  SaturateOnIntegerOverflow=off
  Abs1 : Abs  SaturateOnIntegerOverflow=off
  Abs2 : Abs  SaturateOnIntegerOverflow=off
  Add : Sum
  Add1 : Sum  Inputs=+-
  Add2 : Sum  Inputs=++++
  CDmin : Constant  Value=CDmin
  CL_CDmin : Constant  Value=CL_CDmin
  CdDa : Constant  Value=CdDa
  CdDe : Constant  Value=CdDe
  CdDr : Constant  Value=CdDr
  Constant1 : Constant  Value=K
  Gain : Gain  Gain=-1
  Product{,2..4} (4 alike) : Product
  Square : Math  Operator=square
  CD : Outport
  wires:
  CDmin/1 -> Add/1
  CL/1 -> Add1/1
  CL_CDmin/1 -> Add1/2
  Add1/1 -> Square/1
  Square/1 -> Product/2
  Constant1/1 -> Product/1
  Product/1 -> Add/2
  Add/1 -> Add2/1
  aileron/1 -> Abs/1
  Abs/1 -> Product2/1
  CdDa/1 -> Product2/2
  Product2/1 -> Add2/2
  Abs1/1 -> Product3/1
  rudder/1 -> Abs1/1
  CdDr/1 -> Product3/2
  elevator/1 -> Abs2/1
  Abs2/1 -> Product4/1
  CdDe/1 -> Product4/2
  Product3/1 -> Add2/3
  Product4/1 -> Add2/4
  Add2/1 -> Gain/1
  Gain/1 -> CD/1

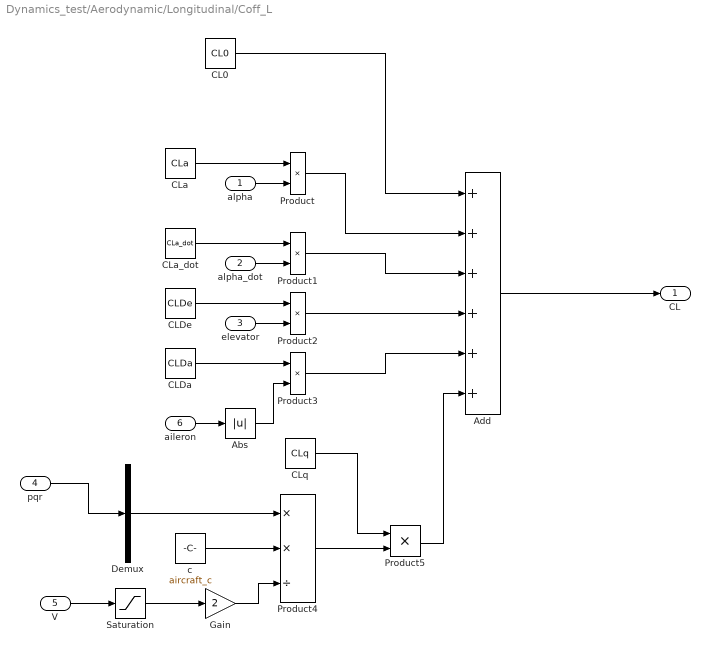
== system Dynamics_test/Aerodynamic/Longitudinal/Coff_L ==
  alpha : Inport
  alpha_dot : Inport  Port=2
  elevator : Inport  Port=3
  pqr : Inport  Port=4
  V : Inport  Port=5
  aileron : Inport  Port=6
  Abs : Abs  SaturateOnIntegerOverflow=off
  Add : Sum  Inputs=++++++
  CL0 : Constant  Value=CL0
  CLDa : Constant  Value=CLDa
  CLDe : Constant  Value=CLDe
  CLa : Constant  Value=CLa
  CLa_dot : Constant  Value=CLa_dot
  CLq : Constant  Value=CLq
  Demux : Demux  Outputs=3
  Gain : Gain  Gain=2
  Product{,1..3,5} (5 alike) : Product
  Product4 : Product  Inputs=**/
  Saturation : Saturate  UpperLimit=inf  LowerLimit=0.1
  c : Constant  Value=aircraft_c
  CL : Outport
  wires:
  alpha/1 -> Product/2
  CLa/1 -> Product/1
  CL0/1 -> Add/1
  Product/1 -> Add/2
  CLa_dot/1 -> Product1/1
  alpha_dot/1 -> Product1/2
  Product1/1 -> Add/3
  elevator/1 -> Product2/2
  CLDe/1 -> Product2/1
  Product2/1 -> Add/4
  CLDa/1 -> Product3/1
  Product3/1 -> Add/5
  aileron/1 -> Abs/1
  Abs/1 -> Product3/2
  pqr/1 -> Demux/1
  Demux/2 -> Product4/1
  c/1 -> Product4/2
  V/1 -> Saturation/1
  Saturation/1 -> Gain/1
  Gain/1 -> Product4/3
  CLq/1 -> Product5/1
  Product4/1 -> Product5/2
  Product5/1 -> Add/6
  Add/1 -> CL/1

== system Dynamics_test/Aerodynamic/Longitudinal/Subsystem ==
  alpha : Inport
  elevator : Inport  Port=2
  pqr : Inport  Port=3
  V : Inport  Port=4
  Add : Sum  Inputs=++++
  Cm0 : Constant  Value=Cm0
  CmDe : Constant  Value=CmDe
  Cma : Constant  Value=Cma
  Cmq : Constant  Value=Cmq
  Demux : Demux  Outputs=3
  Gain : Gain  Gain=2
  Product : Product
  Product1 : Product
  Product4 : Product  Inputs=**/
  Product5 : Product
  Saturation : Saturate  UpperLimit=inf  LowerLimit=0.1
  c : Constant  Value=aircraft_c
  Cm : Outport
  wires:
  Cm0/1 -> Add/1
  alpha/1 -> Product/2
  Cma/1 -> Product/1
  Product/1 -> Add/2
  elevator/1 -> Product1/2
  CmDe/1 -> Product1/1
  Product1/1 -> Add/3
  Saturation/1 -> Gain/1
  Cmq/1 -> Product5/1
  Gain/1 -> Product4/3
  V/1 -> Saturation/1
  Product4/1 -> Product5/2
  c/1 -> Product4/2
  Demux/2 -> Product4/1
  pqr/1 -> Demux/1
  Product5/1 -> Add/4
  Add/1 -> Cm/1

== system Dynamics_test/Aerodynamic/Lateral/Coff_CY/roll//yaw factors ==
  pqr : Inport
  V : Inport  Port=2
  Cmq : Constant
  Coff_Yp : Constant  Value=CYp
  Coff_Yr : Constant  Value=CYr
  Demux : Demux  Outputs=3
  Gain : Gain  Gain=2
  Product : Product  Inputs=***/
  Product1 : Product
  Product2 : Product  Inputs=***/
  Product3 : Product
  Saturation : Saturate  UpperLimit=inf  LowerLimit=0.1
  b : Constant  Value=aircraft_b
  CYp : Outport
  CYr : Outport  Port=2
  wires:
  pqr/1 -> Demux/1
  Demux/1 -> Product/1
  Cmq/1 -> Product2/2, Product/2
  b/1 -> Product2/3, Product/3
  V/1 -> Saturation/1
  Saturation/1 -> Gain/1
  Gain/1 -> Product2/4, Product/4
  Product1/1 -> CYp/1
  Product/1 -> Product1/2
  Coff_Yp/1 -> Product1/1
  Product2/1 -> Product3/1
  Coff_Yr/1 -> Product3/2
  Demux/3 -> Product2/1
  Product3/1 -> CYr/1

== system Dynamics_test/Aerodynamic/Lateral/Coff_Cl/roll//yaw factors ==
  pqr : Inport
  V : Inport  Port=2
  Cmq : Constant  Value=0.5
  Coff_lp : Constant  Value=Clp
  Coff_lr : Constant  Value=Clr
  Demux : Demux  Outputs=3
  Product : Product  Inputs=***/
  Product1 : Product
  Product2 : Product  Inputs=***/
  Product3 : Product
  Saturation : Saturate  UpperLimit=inf  LowerLimit=0.1
  b : Constant  Value=aircraft_b
  Clp : Outport
  Clr : Outport  Port=2
  wires:
  pqr/1 -> Demux/1
  Product/1 -> Product1/2
  Cmq/1 -> Product2/2, Product/2
  b/1 -> Product2/3, Product/3
  Demux/1 -> Product/1
  V/1 -> Saturation/1
  Saturation/1 -> Product2/4, Product/4
  Product1/1 -> Clp/1
  Coff_lp/1 -> Product1/1
  Demux/3 -> Product2/1
  Product2/1 -> Product3/1
  Coff_lr/1 -> Product3/2
  Product3/1 -> Clr/1

== system Dynamics_test/Aerodynamic/Lateral/Subsystem/roll//yaw factors ==
  pqr : Inport
  V : Inport  Port=2
  Cmq : Constant  Value=0.5
  Coff_np : Constant  Value=Cnp
  Coff_nr : Constant  Value=Cnr
  Demux : Demux  Outputs=3
  Product : Product  Inputs=***/
  Product1 : Product
  Product2 : Product  Inputs=***/
  Product3 : Product
  Saturation : Saturate  UpperLimit=inf  LowerLimit=0.1
  b : Constant  Value=aircraft_b
  Cnp : Outport
  Cnr : Outport  Port=2
  wires:
  pqr/1 -> Demux/1
  Product/1 -> Product1/2
  Cmq/1 -> Product2/2, Product/2
  b/1 -> Product2/3, Product/3
  Demux/1 -> Product/1
  V/1 -> Saturation/1
  Saturation/1 -> Product2/4, Product/4
  Product1/1 -> Cnp/1
  Coff_np/1 -> Product1/1
  Demux/3 -> Product2/1
  Product2/1 -> Product3/1
  Coff_nr/1 -> Product3/2
  Product3/1 -> Cnr/1
